simulink model "dyn_graph_sim_compact"  (R2022b)
settings: Solver=VariableStepAuto  StartTime=0.0  StopTime=100  RelTol=1e-3
values from neighbouring files (symbols this model uses):
  A = [0 1 0; 0 0 1; 0 0 -1/tau]    [cacc_consensus_main.m]    (also in dyn_graph.m; dyn_graph_10.m; dyn_graph_10_disturb.m; fixed_graph.m)
  B = [0 0 1/tau]'    [cacc_consensus_main.m]    (also in dyn_graph.m; dyn_graph_10.m; dyn_graph_10_disturb.m; fixed_graph.m)
  C = diag([1 1 1])    [cacc_consensus_main.m]    (also in dyn_graph.m; dyn_graph_10.m; dyn_graph_10_disturb.m; fixed_graph.m)
  D = [0 0 0]'    [cacc_consensus_main.m]    (also in dyn_graph.m; dyn_graph_10.m; dyn_graph_10_disturb.m; fixed_graph.m)
  h = 1    [cacc_consensus_main.m]    (also in dyn_graph.m; dyn_graph_10.m; dyn_graph_10_disturb.m; fixed_graph.m)
  K_cacc1 = [2.3231, 2.3783, -0.3394]    [dyn_graph.m]    (also in dyn_graph_10.m = -K_lmi; dyn_graph_10_disturb.m = -K_lmi; string_stability_test.m)
  K_cacc2 = [ 19.3466, 17.8329, 1.8423]    [dyn_graph.m]    (also in dyn_graph_10.m = -K_lmi; dyn_graph_10_disturb.m = -K_lmi)
  L1 = [0 0 0 0 ... (first row only)    [dyn_graph.m]    (also in dyn_graph_10.m = [0 0 0 0 0 0 0 0 0 0 0; dyn_graph_10_disturb.m = [0 0 0 0 0 0 0 0 0 0 0)
  L2 = [0 0 0 0 ... (first row only)    [dyn_graph.m]    (also in dyn_graph_10.m = [0 0 0 0 0 0 0 0 0 0 0; dyn_graph_10_disturb.m = [0 0 0 0 0 0 0 0 0 0 0)
  lv = 4.46    [cacc_consensus_main.m]    (also in dyn_graph.m; dyn_graph_10.m; dyn_graph_10_disturb.m; fixed_graph.m)
  q0_init = 0    [cacc_consensus_main.m]    (also in dyn_graph.m; dyn_graph_10.m = rand() * range; dyn_graph_10_disturb.m = rand() * range; fixed_graph.m = rand() * range)
  q1_init = 0    [cacc_consensus_main.m]    (also in dyn_graph.m; dyn_graph_10.m = rand() * range; dyn_graph_10_disturb.m = rand() * range; fixed_graph.m = rand() * range)
  q2_init = 0    [cacc_consensus_main.m]    (also in dyn_graph.m; dyn_graph_10.m = rand() * range; dyn_graph_10_disturb.m = rand() * range; fixed_graph.m = rand() * range)
  q3_init = 0    [cacc_consensus_main.m]    (also in dyn_graph.m; dyn_graph_10.m = rand() * range; dyn_graph_10_disturb.m = rand() * range; fixed_graph.m = rand() * range)
  q4_init = rand() * range    [dyn_graph_10.m]    (also in dyn_graph_10_disturb.m; fixed_graph.m; fixed_graph_lpv.m)
  q5_init = rand() * range    [dyn_graph_10.m]    (also in dyn_graph_10_disturb.m; fixed_graph.m; fixed_graph_lpv.m)
  q6_init = rand() * range    [dyn_graph_10.m]    (also in dyn_graph_10_disturb.m; fixed_graph.m; fixed_graph_lpv.m)
  q7_init = rand() * range    [dyn_graph_10.m]    (also in dyn_graph_10_disturb.m; fixed_graph.m; fixed_graph_lpv.m)
  rv = 0    [cacc_consensus_main.m]    (also in dyn_graph.m; dyn_graph_10.m; dyn_graph_10_disturb.m; fixed_graph.m)
  tau = 0.1    [cacc_consensus_main.m]    (also in dyn_graph.m; dyn_graph_10.m; dyn_graph_10_disturb.m; fixed_graph.m)
libraries: cstblocks x11, simulink x2
settings Model: Creator=phatdo  LastModifiedBy=phatdo
settings DataIOCC: ReturnWorkspaceOutputs=off

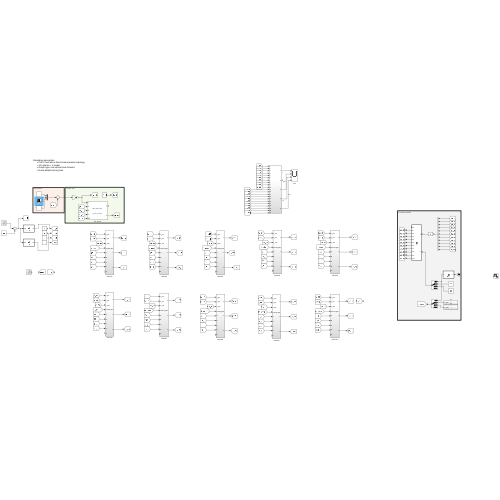
[thumbnail: Simulink's stored preview of the top-level diagram]
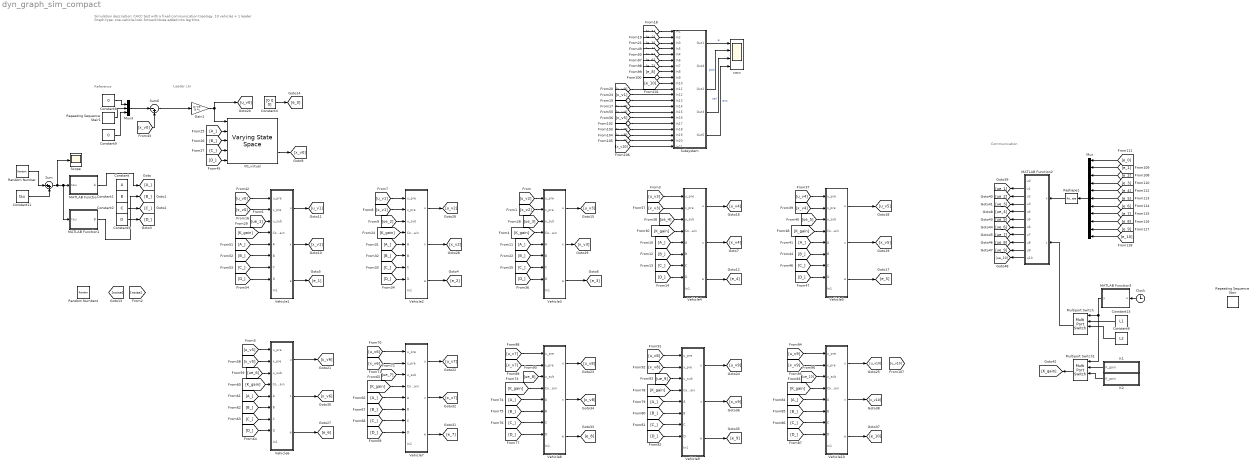
== system dyn_graph_sim_compact ==
  note: Reference
  note: Leader car
  note: Simulation description:
      | CACC test with a fixed communication topology.
      | 10 vehicles + 1 leader
      | Graph type: one-vehicle-look-forward
      | Noise added into lag time
  note: Communication
  Clock : Clock
  Constant : Constant  Value=A
  Constant1 : Constant  Value=B
  Constant11 : Constant  Value=tau
  Constant13 : Constant  Value=L1
  Constant2 : Constant  Value=C
  Constant3 : Constant  Value=D
  Constant4 : Constant  Value=[0 0 0]
  Constant6 : Constant  Value=L2
  Constant8 : Constant  Value=0
  Constant9 : Constant  Value=0
  Gain1 : Gain  Gain=[0 -0.5 0]  Multiplication=Matrix(K*u) (u vector)
  K1 : Subsystem
  K2 : Subsystem
  MATLAB Function : MATLAB Function  TreatAsAtomicUnit=on
  MATLAB Function1 : MATLAB Function  TreatAsAtomicUnit=on
  MATLAB Function2 : MATLAB Function  TreatAsAtomicUnit=on
  MATLAB Function3 : MATLAB Function  TreatAsAtomicUnit=on
  Multiport Switch : MultiPortSwitch  SaturateOnIntegerOverflow=off  InputSameDT=off
  Multiport Switch1 : MultiPortSwitch  SaturateOnIntegerOverflow=off  InputSameDT=off
  Mux : Mux  Inputs=11
  Mux3 : Mux  Inputs=3
  Random Number : RandomNumber  Variance=0.0001  SampleTime=0.1
  Random Number4 : RandomNumber  Variance=0.1  SampleTime=0.1
  Repeating Sequence Stair : simulink/Sources/Repeating Sequence Stair  OutValues=[2 1].'  tsamp=30  OutMin=[]  OutMax=[]  OutDataTypeStr=double  OutputDataTypeScalingMode=double  OutDataType=fixdt(0,8)  ConRadixGroup=Best Precision: Vector-wise  OutScaling=2^-12
  Repeating Sequence Stair1 : simulink/Sources/Repeating Sequence Stair  OutValues=[5 5 5 25 25 25 5 5 5 5]  tsamp=10  OutMin=[]  OutMax=[]  OutDataTypeStr=double  OutputDataTypeScalingMode=double  OutDataType=fixdt(0,8)  ConRadixGroup=Best Precision: Vector-wise  OutScaling=2^-12
  Reshape1 : Reshape  OutputDimensionality=Customize  OutputDimensions=[3,11]
  Scope : Scope
  Subsystem : Subsystem
  Sum : Sum  Inputs=|++
  Sum6 : Sum  Inputs=|-+
  V0_virtual : cstblocks/Linear Parameter Varying/Varying State Space  x0=[q0_init;0;0]  xNames=''  OutputX=on  OutputDX=off
  Vehicle1 : Subsystem
  Vehicle10 : Subsystem
  Vehicle2 : Subsystem
  Vehicle3 : Subsystem
  Vehicle4 : Subsystem
  Vehicle5 : Subsystem
  Vehicle6 : Subsystem
  Vehicle7 : Subsystem
  Vehicle8 : Subsystem
  Vehicle9 : Subsystem
  cacc : Scope  NumInputPorts=4
  wires:
  Constant2/1 -> [C_]
  Constant3/1 -> [D_]
  Repeating Sequence Stair1/1 -> Mux3/2
  [D_] -> V0_virtual/5
  V0_virtual/2 -> [x_v0]
  [B_] -> V0_virtual/3
  [A_] -> V0_virtual/2
  Constant9/1 -> Mux3/3
  Constant8/1 -> Mux3/1
  [x_v0] -> Sum6/2
  [C_] -> V0_virtual/4
  Sum6/1 -> Gain1/1
  Gain1/1 -> V0_virtual/1, [u_v0]
  Mux3/1 -> Sum6/1
  Sum/1 -> Scope/1, MATLAB Function1/1(tau), MATLAB Function/1(tau)
  Constant11/1 -> Sum/2
  Random Number/1 -> Sum/1
  MATLAB Function/1(A) -> [A_]
  MATLAB Function1/1(B) -> [B_]
  [u_v0] -> Vehicle1/1(u_pre)
  [K_gain] -> Vehicle1/4(Control gain)
  [A_] -> Vehicle1/5(A)
  [B_] -> Vehicle1/6(B)
  [C_] -> Vehicle1/7(C)
  [x_v0] -> Vehicle1/2(x_pre)
  [D_] -> Vehicle1/8(D)
  Vehicle1/1(u) -> [u_v1]
  Vehicle1/2(x) -> [x_v1]
  Vehicle1/3(e) -> [e_1]
  Constant4/1 -> [e_0]
  [u_v1] -> Vehicle2/1(u_pre)
  [x_v1] -> Vehicle2/2(x_pre)
  Vehicle2/3(e) -> [e_2]
  Vehicle2/2(x) -> [x_v2]
  Vehicle2/1(u) -> [u_v2]
  [K_gain] -> Vehicle2/4(Control gain)
  [A_] -> Vehicle2/5(A)
  [B_] -> Vehicle2/6(B)
  [C_] -> Vehicle2/7(C)
  [D_] -> Vehicle2/8(D)
  Vehicle3/2(x) -> [x_v3]
  [u_v2] -> Vehicle3/1(u_pre)
  [x_v2] -> Vehicle3/2(x_pre)
  Vehicle3/3(e) -> [e_3]
  [K_gain] -> Vehicle3/4(Control gain)
  [A_] -> Vehicle3/5(A)
  [B_] -> Vehicle3/6(B)
  [C_] -> Vehicle3/7(C)
  [D_] -> Vehicle3/8(D)
  Vehicle4/2(x) -> [x_v4]
  [u_v3] -> Vehicle4/1(u_pre)
  [x_v3] -> Vehicle4/2(x_pre)
  [B_] -> Vehicle4/6(B)
  [K_gain] -> Vehicle4/4(Control gain)
  [D_] -> Vehicle4/8(D)
  Vehicle4/3(e) -> [e_4]
  [C_] -> Vehicle4/7(C)
  [A_] -> Vehicle4/5(A)
  Vehicle3/1(u) -> [u_v3]
  Vehicle4/1(u) -> [u_v4]
  [u_v4] -> Vehicle5/1(u_pre)
  [x_v4] -> Vehicle5/2(x_pre)
  Vehicle5/3(e) -> [e_5]
  [K_gain] -> Vehicle5/4(Control gain)
  [A_] -> Vehicle5/5(A)
  [B_] -> Vehicle5/6(B)
  [C_] -> Vehicle5/7(C)
  [D_] -> Vehicle5/8(D)
  Vehicle5/2(x) -> [x_v5]
  Vehicle6/1(u) -> [u_v6]
  Vehicle7/1(u) -> [u_v7]
  Vehicle5/1(u) -> [u_v5]
  Vehicle8/1(u) -> [u_v8]
  Vehicle9/1(u) -> [u_v9]
  Vehicle10/1(u) -> [u_v10]
  [u_v5] -> Vehicle6/1(u_pre)
  [x_v5] -> Vehicle6/2(x_pre)
  Vehicle6/3(e) -> [e_6]
  Vehicle6/2(x) -> [x_v6]
  [K_gain] -> Vehicle6/4(Control gain)
  [A_] -> Vehicle6/5(A)
  [B_] -> Vehicle6/6(B)
  [C_] -> Vehicle6/7(C)
  [D_] -> Vehicle6/8(D)
  [K_gain] -> Vehicle7/4(Control gain)
  [A_] -> Vehicle7/5(A)
  [B_] -> Vehicle7/6(B)
  [C_] -> Vehicle7/7(C)
  [D_] -> Vehicle7/8(D)
  [u_v6] -> Vehicle7/1(u_pre)
  [x_v6] -> Vehicle7/2(x_pre)
  Vehicle7/3(e) -> [e_7]
  Vehicle7/2(x) -> [x_v7]
  Vehicle8/2(x) -> [x_v8]
  Vehicle9/2(x) -> [x_v9]
  Vehicle10/2(x) -> [x_v10]
  Vehicle10/3(e) -> [e_10]
  Vehicle9/3(e) -> [e_9]
  Vehicle8/3(e) -> [e_8]
  [K_gain] -> Vehicle8/4(Control gain)
  [A_] -> Vehicle8/5(A)
  [B_] -> Vehicle8/6(B)
  [C_] -> Vehicle8/7(C)
  [D_] -> Vehicle8/8(D)
  [K_gain] -> Vehicle9/4(Control gain)
  [A_] -> Vehicle9/5(A)
  [B_] -> Vehicle9/6(B)
  [C_] -> Vehicle9/7(C)
  [D_] -> Vehicle9/8(D)
  [K_gain] -> Vehicle10/4(Control gain)
  [A_] -> Vehicle10/5(A)
  [B_] -> Vehicle10/6(B)
  [C_] -> Vehicle10/7(C)
  [D_] -> Vehicle10/8(D)
  [u_v7] -> Vehicle8/1(u_pre)
  [x_v7] -> Vehicle8/2(x_pre)
  [u_v8] -> Vehicle9/1(u_pre)
  [x_v8] -> Vehicle9/2(x_pre)
  [u_v9] -> Vehicle10/1(u_pre)
  [x_v9] -> Vehicle10/2(x_pre)
  Multiport Switch1/1 -> [K_gain]
  MATLAB Function2/3(u2) -> [ue_2]
  [e_2] -> Mux/3
  [e_1] -> Mux/2
  Reshape1/1 -> MATLAB Function2/1(x)
  [e_0] -> Mux/1
  Multiport Switch/1 -> MATLAB Function2/2(L)
  Constant6/1 -> Multiport Switch/3
  Constant13/1 -> Multiport Switch/2
  Mux/1 -> Reshape1/1
  MATLAB Function2/2(u1) -> [ue_1]
  MATLAB Function2/4(u3) -> [ue_3]
  [e_3] -> Mux/4
  MATLAB Function2/5(u4) -> [ue_4]
  MATLAB Function2/6(u5) -> [ue_5]
  MATLAB Function2/7(u6) -> [ue_6]
  MATLAB Function2/8(u7) -> [ue_7]
  MATLAB Function2/9(u8) -> [ue_8]
  MATLAB Function2/10(u9) -> [ue_9]
  MATLAB Function2/11(u10) -> [ue_10]
  [e_4] -> Mux/5
  [e_5] -> Mux/6
  [e_6] -> Mux/7
  [e_7] -> Mux/8
  [e_8] -> Mux/9
  [e_9] -> Mux/10
  [e_10] -> Mux/11
  [ue_10] -> Vehicle10/3(u_sub)
  [ue_9] -> Vehicle9/3(u_sub)
  [ue_8] -> Vehicle8/3(u_sub)
  [ue_7] -> Vehicle7/3(u_sub)
  [ue_6] -> Vehicle6/3(u_sub)
  [ue_5] -> Vehicle5/3(u_sub)
  [ue_4] -> Vehicle4/3(u_sub)
  [ue_3] -> Vehicle3/3(u_sub)
  [ue_2] -> Vehicle2/3(u_sub)
  [ue_1] -> Vehicle1/3(u_sub)
  Clock/1 -> MATLAB Function3/1(u)
  MATLAB Function3/1(y) -> Multiport Switch1/1, Multiport Switch/1
  K1/1(K_gain) -> Multiport Switch1/2
  K2/1(K_gain) -> Multiport Switch1/3
  [x_v0] -> Subsystem/11(In11)
  [x_v5] -> Subsystem/16(In16)
  [x_v9] -> Subsystem/20(In20)
  Subsystem/1(Out1) -> cacc/1  "e"
  [x_v10] -> Subsystem/21(In21)
  [e_10] -> Subsystem/10(In10)
  [e_9] -> Subsystem/9(In9)
  [e_7] -> Subsystem/7(In7)
  [e_6] -> Subsystem/6(In6)
  [x_v8] -> Subsystem/19(In19)
  [e_8] -> Subsystem/8(In8)
  [x_v7] -> Subsystem/18(In18)
  [x_v2] -> Subsystem/13(In13)
  [e_1] -> Subsystem/1(In1)
  [x_v6] -> Subsystem/17(In17)
  [e_4] -> Subsystem/4(In5)
  [x_v3] -> Subsystem/14(In14)
  Subsystem/5(Out5) -> cacc/4  "acc"
  [x_v1] -> Subsystem/12(In12)
  Subsystem/4(Out3) -> cacc/3  "vel"
  [e_3] -> Subsystem/3(In3)
  Subsystem/3(Out2) -> cacc/2  "pos"
  [e_5] -> Subsystem/5(In4)
  [x_v4] -> Subsystem/15(In15)
  [e_2] -> Subsystem/2(In2)

== system dyn_graph_sim_compact/K1 ==
  Constant : Constant
  K1 : Fcn  Expr=-K_cacc1(2)
  K2 : Fcn  Expr=0
  K4 : Fcn  Expr=-K_cacc1(1)
  Mux : Mux  Inputs=3
  Reshape : Reshape  OutputDimensionality=Customize  OutputDimensions=[1,3]
  K_gain : Outport
  wires:
  Mux/1 -> Reshape/1
  Reshape/1 -> K_gain/1
  K4/1 -> Mux/1
  K1/1 -> Mux/2
  K2/1 -> Mux/3
  Constant/1 -> K2/1, K1/1, K4/1

== system dyn_graph_sim_compact/K2 ==
  Constant : Constant
  K1 : Fcn  Expr=-K_cacc2(2)
  K2 : Fcn  Expr=0
  K4 : Fcn  Expr=-K_cacc2(1)
  Mux : Mux  Inputs=3
  Reshape : Reshape  OutputDimensionality=Customize  OutputDimensions=[1,3]
  K_gain : Outport
  wires:
  Mux/1 -> Reshape/1
  Reshape/1 -> K_gain/1
  K4/1 -> Mux/1
  K1/1 -> Mux/2
  K2/1 -> Mux/3
  Constant/1 -> K2/1, K1/1, K4/1

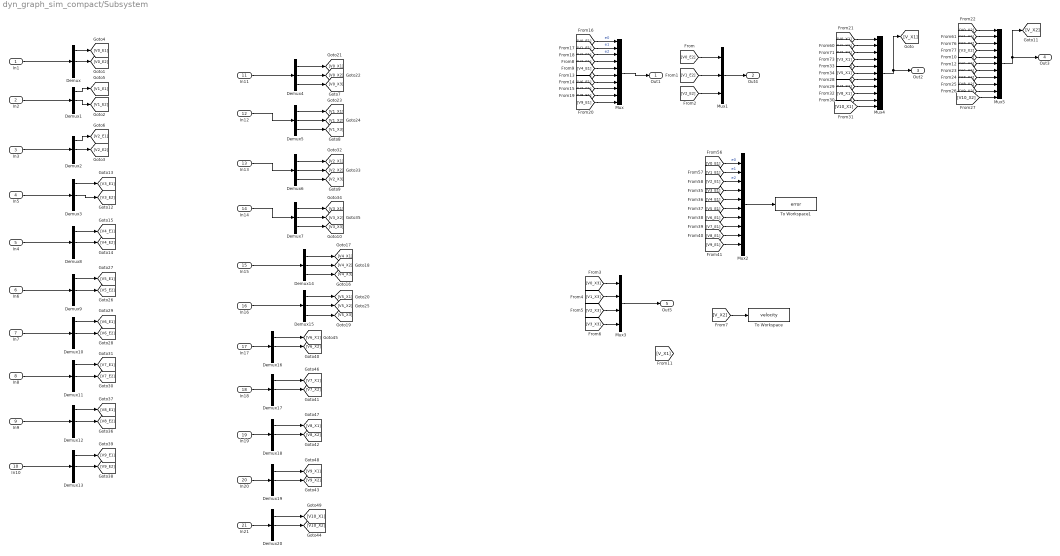
== system dyn_graph_sim_compact/Subsystem ==
  In1 : Inport
  In2 : Inport  Port=2
  In3 : Inport  Port=3
  In5 : Inport  Port=4
  In4 : Inport  Port=5
  In6 : Inport  Port=6
  In7 : Inport  Port=7
  In8 : Inport  Port=8
  In9 : Inport  Port=9
  In10 : Inport  Port=10
  In11 : Inport  Port=11
  In12 : Inport  Port=12
  In13 : Inport  Port=13
  In14 : Inport  Port=14
  In15 : Inport  Port=15
  In16 : Inport  Port=16
  In17 : Inport  Port=17
  In18 : Inport  Port=18
  In19 : Inport  Port=19
  In20 : Inport  Port=20
  In21 : Inport  Port=21
  Demux{,1..20} (21 alike) : Demux  Outputs=3
  Mux : Mux  Inputs=10
  Mux1 : Mux  Inputs=3
  Mux2 : Mux  Inputs=10
  Mux3 : Mux
  Mux4 : Mux  Inputs=11
  Mux5 : Mux  Inputs=11
  To Workspace : ToWorkspace  VariableName=velocity  SaveFormat=Timeseries  SampleTime=-1
  To Workspace1 : ToWorkspace  VariableName=error  SaveFormat=Timeseries  SampleTime=-1
  Out1 : Outport
  Out4 : Outport  Port=2
  Out2 : Outport  Port=3
  Out3 : Outport  Port=4
  Out5 : Outport  Port=5
  wires:
  [V2_X1] -> Mux4/3
  Demux/1 -> [V0_E1]
  Demux2/1 -> [V2_E1]
  In2/1 -> Demux1/1
  [V0_X1] -> Mux4/1
  Demux1/1 -> [V1_E1]
  [V3_X1] -> Mux4/4
  Demux6/2 -> [V2_X2]
  Demux7/1 -> [V3_X1]
  Demux4/1 -> [V0_X1]
  Demux4/2 -> [V0_X2]
  Demux5/2 -> [V1_X2]
  Demux6/1 -> [V2_X1]
  [V1_X2] -> Mux5/2
  In1/1 -> Demux/1
  Mux4/1 -> [V_X1], Out2/1
  [V3_X2] -> Mux5/4
  [V2_X2] -> Mux5/3
  [V0_X2] -> Mux5/1
  Demux7/2 -> [V3_X2]
  [V1_E1] -> Mux/2  "e1"
  [V1_X1] -> Mux4/2
  [V2_E1] -> Mux/3  "e2"
  [V0_E1] -> Mux/1  "e0"
  Mux/1 -> Out1/1
  In3/1 -> Demux2/1
  Demux5/1 -> [V1_X1]
  Demux/2 -> [V0_E2]
  Demux1/2 -> [V1_E2]
  Demux2/2 -> [V2_E2]
  [V0_E2] -> Mux1/1
  [V1_E2] -> Mux1/2
  [V2_E2] -> Mux1/3
  Mux1/1 -> Out4/1
  Demux4/3 -> [V0_X3]
  Demux5/3 -> [V1_X3]
  Demux6/3 -> [V2_X3]
  Demux7/3 -> [V3_X3]
  [V0_X3] -> Mux3/1
  [V1_X3] -> Mux3/2
  [V2_X3] -> Mux3/3
  [V3_X3] -> Mux3/4
  Mux3/1 -> Out5/1
  Mux5/1 -> [V_X2], Out3/1
  In5/1 -> Demux3/1
  In4/1 -> Demux8/1
  In6/1 -> Demux9/1
  In7/1 -> Demux10/1
  In8/1 -> Demux11/1
  In9/1 -> Demux12/1
  In10/1 -> Demux13/1
  In11/1 -> Demux4/1
  In12/1 -> Demux5/1
  In13/1 -> Demux6/1
  In14/1 -> Demux7/1
  Demux3/1 -> [V3_E1]
  Demux8/1 -> [V4_E1]
  Demux3/2 -> [V3_E2]
  Demux8/2 -> [V4_E2]
  Demux14/1 -> [V4_X1]
  In15/1 -> Demux14/1
  Demux14/2 -> [V4_X2]
  Demux14/3 -> [V4_X3]
  Demux15/1 -> [V5_X1]
  In16/1 -> Demux15/1
  Demux15/2 -> [V5_X2]
  Demux15/3 -> [V5_X3]
  [V3_E1] -> Mux/4
  [V4_E1] -> Mux/5
  [V4_X2] -> Mux5/5
  [V5_X2] -> Mux5/6
  Demux9/1 -> [V5_E1]
  Demux9/2 -> [V5_E2]
  Demux10/1 -> [V6_E1]
  Demux10/2 -> [V6_E2]
  Demux11/1 -> [V7_E1]
  Demux11/2 -> [V7_E2]
  Demux12/1 -> [V8_E1]
  Demux12/2 -> [V8_E2]
  Demux13/1 -> [V9_E1]
  Demux13/2 -> [V9_E2]
  [V5_E1] -> Mux/6
  [V6_E1] -> Mux/7
  [V7_E1] -> Mux/8
  [V8_E1] -> Mux/9
  [V9_E1] -> Mux/10
  Demux16/2 -> [V6_X2]
  Demux17/2 -> [V7_X2]
  Demux18/2 -> [V8_X2]
  Demux19/2 -> [V9_X2]
  Demux20/2 -> [V10_X2]
  In17/1 -> Demux16/1
  In18/1 -> Demux17/1
  In19/1 -> Demux18/1
  In20/1 -> Demux19/1
  In21/1 -> Demux20/1
  [V6_X2] -> Mux5/7
  [V7_X2] -> Mux5/8
  [V8_X2] -> Mux5/9
  [V9_X2] -> Mux5/10
  [V10_X2] -> Mux5/11
  Demux16/1 -> [V6_X1]
  Demux17/1 -> [V7_X1]
  Demux18/1 -> [V8_X1]
  Demux19/1 -> [V9_X1]
  Demux20/1 -> [V10_X1]
  [V4_X1] -> Mux4/5
  [V5_X1] -> Mux4/6
  [V6_X1] -> Mux4/7
  [V7_X1] -> Mux4/8
  [V8_X1] -> Mux4/9
  [V9_X1] -> Mux4/10
  [V10_X1] -> Mux4/11
  [V_X2] -> To Workspace/1
  [V0_E1] -> Mux2/1  "e0"
  [V1_E1] -> Mux2/2  "e1"
  [V2_E1] -> Mux2/3  "e2"
  [V3_E1] -> Mux2/4
  [V4_E1] -> Mux2/5
  [V5_E1] -> Mux2/6
  [V6_E1] -> Mux2/7
  [V7_E1] -> Mux2/8
  [V8_E1] -> Mux2/9
  [V9_E1] -> Mux2/10
  Mux2/1 -> To Workspace1/1

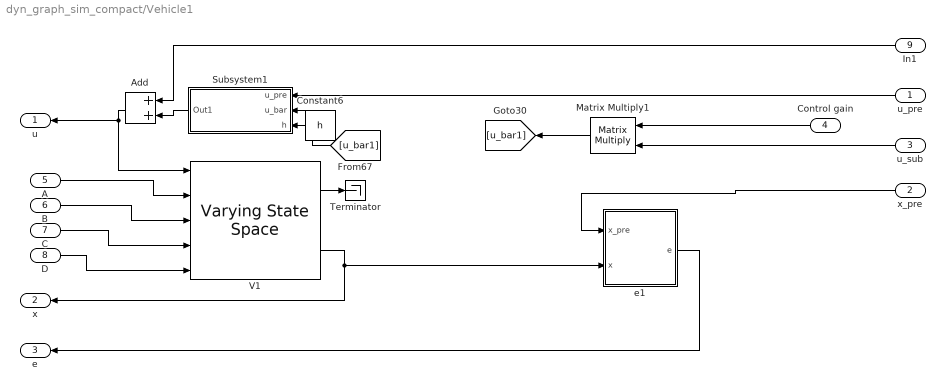
== system dyn_graph_sim_compact/Vehicle1 ==
  u_pre : Inport
  x_pre : Inport  Port=2
  u_sub : Inport  Port=3
  Control gain : Inport  Port=4
  A : Inport  Port=5
  B : Inport  Port=6
  C : Inport  Port=7
  D : Inport  Port=8
  In1 : Inport  Port=9
  Add : Sum
  Constant6 : Constant  Value=h
  Matrix Multiply1 : Product  Multiplication=Matrix(*)
  Subsystem1 : Subsystem
  Terminator : Terminator
  V1 : cstblocks/Linear Parameter Varying/Varying State Space  x0=[q1_init;0;0]  xNames=''  OutputX=on  OutputDX=off
  e1 : Subsystem
  u : Outport
  x : Outport  Port=2
  e : Outport  Port=3
  wires:
  C/1 -> V1/4
  Matrix Multiply1/1 -> [u_bar1]
  Constant6/1 -> Subsystem1/3(h)
  x_pre/1 -> e1/1(x_pre)
  e1/1(e) -> e/1
  Control gain/1 -> Matrix Multiply1/1
  D/1 -> V1/5
  B/1 -> V1/3
  A/1 -> V1/2
  In1/1 -> Add/1
  Add/1 -> u/1, V1/1
  V1/1 -> Terminator/1
  V1/2 -> x/1, e1/2(x)
  Subsystem1/1(Out1) -> Add/2
  [u_bar1] -> Subsystem1/2(u_bar)
  u_pre/1 -> Subsystem1/1(u_pre)
  u_sub/1 -> Matrix Multiply1/2

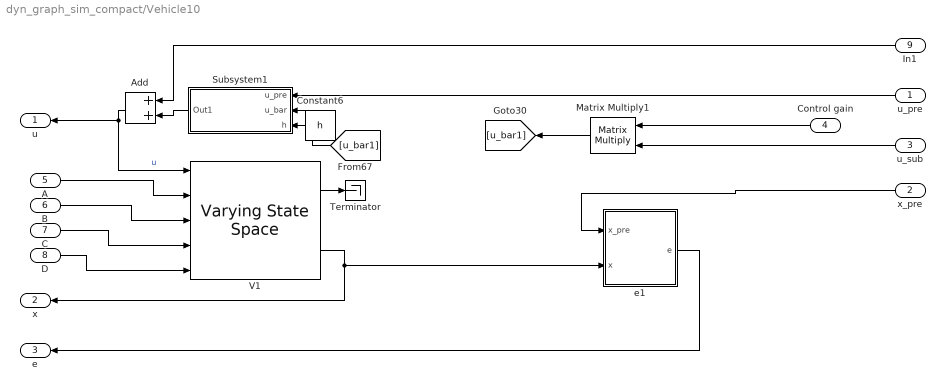
== system dyn_graph_sim_compact/Vehicle10 ==
  u_pre : Inport
  x_pre : Inport  Port=2
  u_sub : Inport  Port=3
  Control gain : Inport  Port=4
  A : Inport  Port=5
  B : Inport  Port=6
  C : Inport  Port=7
  D : Inport  Port=8
  In1 : Inport  Port=9
  Add : Sum
  Constant6 : Constant  Value=h
  Matrix Multiply1 : Product  Multiplication=Matrix(*)
  Subsystem1 : Subsystem
  Terminator : Terminator
  V1 : cstblocks/Linear Parameter Varying/Varying State Space  x0=[q5_init;0;0]  xNames=''  OutputX=on  OutputDX=off
  e1 : Subsystem
  u : Outport
  x : Outport  Port=2
  e : Outport  Port=3
  wires:
  C/1 -> V1/4
  Matrix Multiply1/1 -> [u_bar1]
  Constant6/1 -> Subsystem1/3(h)
  x_pre/1 -> e1/1(x_pre)
  e1/1(e) -> e/1
  Control gain/1 -> Matrix Multiply1/1
  D/1 -> V1/5
  B/1 -> V1/3
  A/1 -> V1/2
  In1/1 -> Add/1
  Add/1 -> u/1, V1/1  "u"
  V1/1 -> Terminator/1
  V1/2 -> x/1, e1/2(x)
  Subsystem1/1(Out1) -> Add/2
  [u_bar1] -> Subsystem1/2(u_bar)
  u_pre/1 -> Subsystem1/1(u_pre)
  u_sub/1 -> Matrix Multiply1/2

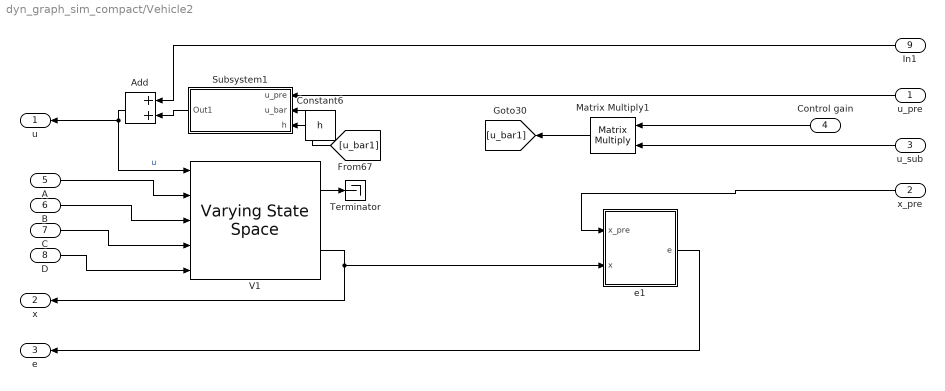
== system dyn_graph_sim_compact/Vehicle2 ==
  u_pre : Inport
  x_pre : Inport  Port=2
  u_sub : Inport  Port=3
  Control gain : Inport  Port=4
  A : Inport  Port=5
  B : Inport  Port=6
  C : Inport  Port=7
  D : Inport  Port=8
  In1 : Inport  Port=9
  Add : Sum
  Constant6 : Constant  Value=h
  Matrix Multiply1 : Product  Multiplication=Matrix(*)
  Subsystem1 : Subsystem
  Terminator : Terminator
  V1 : cstblocks/Linear Parameter Varying/Varying State Space  x0=[q2_init;0;0]  xNames=''  OutputX=on  OutputDX=off
  e1 : Subsystem
  u : Outport
  x : Outport  Port=2
  e : Outport  Port=3
  wires:
  C/1 -> V1/4
  Matrix Multiply1/1 -> [u_bar1]
  Constant6/1 -> Subsystem1/3(h)
  x_pre/1 -> e1/1(x_pre)
  e1/1(e) -> e/1
  Control gain/1 -> Matrix Multiply1/1
  D/1 -> V1/5
  B/1 -> V1/3
  A/1 -> V1/2
  In1/1 -> Add/1
  Add/1 -> u/1, V1/1  "u"
  V1/1 -> Terminator/1
  V1/2 -> x/1, e1/2(x)
  Subsystem1/1(Out1) -> Add/2
  [u_bar1] -> Subsystem1/2(u_bar)
  u_pre/1 -> Subsystem1/1(u_pre)
  u_sub/1 -> Matrix Multiply1/2

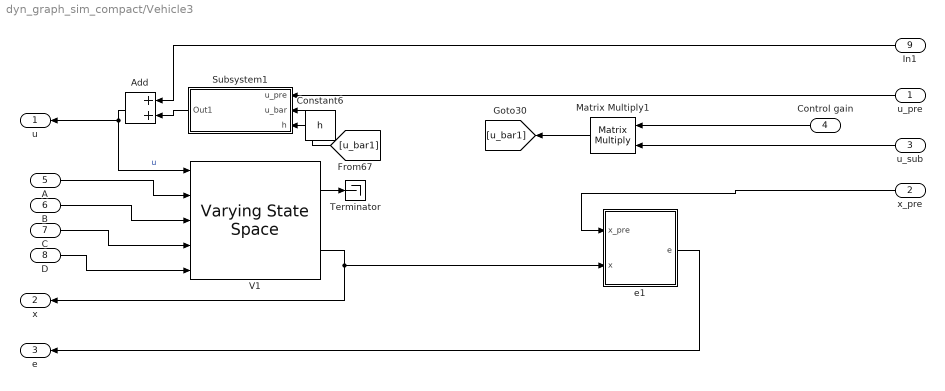
== system dyn_graph_sim_compact/Vehicle3 ==
  u_pre : Inport
  x_pre : Inport  Port=2
  u_sub : Inport  Port=3
  Control gain : Inport  Port=4
  A : Inport  Port=5
  B : Inport  Port=6
  C : Inport  Port=7
  D : Inport  Port=8
  In1 : Inport  Port=9
  Add : Sum
  Constant6 : Constant  Value=h
  Matrix Multiply1 : Product  Multiplication=Matrix(*)
  Subsystem1 : Subsystem
  Terminator : Terminator
  V1 : cstblocks/Linear Parameter Varying/Varying State Space  x0=[q3_init;0;0]  xNames=''  OutputX=on  OutputDX=off
  e1 : Subsystem
  u : Outport
  x : Outport  Port=2
  e : Outport  Port=3
  wires:
  C/1 -> V1/4
  Matrix Multiply1/1 -> [u_bar1]
  Constant6/1 -> Subsystem1/3(h)
  x_pre/1 -> e1/1(x_pre)
  e1/1(e) -> e/1
  Control gain/1 -> Matrix Multiply1/1
  D/1 -> V1/5
  B/1 -> V1/3
  A/1 -> V1/2
  In1/1 -> Add/1
  Add/1 -> u/1, V1/1  "u"
  V1/1 -> Terminator/1
  V1/2 -> x/1, e1/2(x)
  Subsystem1/1(Out1) -> Add/2
  [u_bar1] -> Subsystem1/2(u_bar)
  u_pre/1 -> Subsystem1/1(u_pre)
  u_sub/1 -> Matrix Multiply1/2

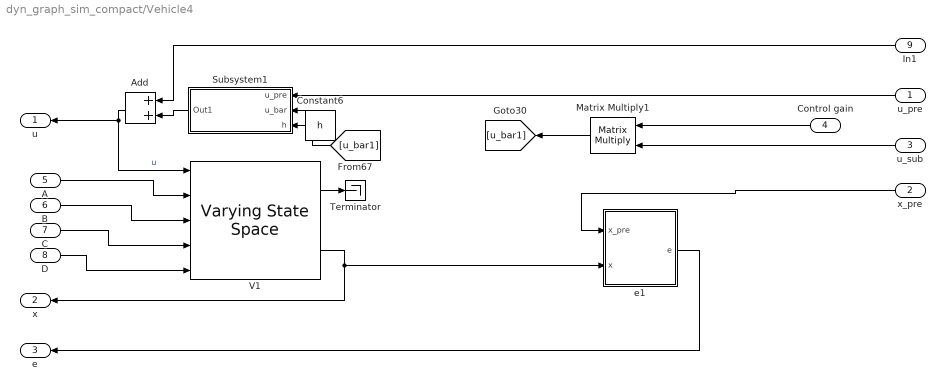
== system dyn_graph_sim_compact/Vehicle4 ==
  u_pre : Inport
  x_pre : Inport  Port=2
  u_sub : Inport  Port=3
  Control gain : Inport  Port=4
  A : Inport  Port=5
  B : Inport  Port=6
  C : Inport  Port=7
  D : Inport  Port=8
  In1 : Inport  Port=9
  Add : Sum
  Constant6 : Constant  Value=h
  Matrix Multiply1 : Product  Multiplication=Matrix(*)
  Subsystem1 : Subsystem
  Terminator : Terminator
  V1 : cstblocks/Linear Parameter Varying/Varying State Space  x0=[q4_init;0;0]  xNames=''  OutputX=on  OutputDX=off
  e1 : Subsystem
  u : Outport
  x : Outport  Port=2
  e : Outport  Port=3
  wires:
  C/1 -> V1/4
  Matrix Multiply1/1 -> [u_bar1]
  Constant6/1 -> Subsystem1/3(h)
  x_pre/1 -> e1/1(x_pre)
  e1/1(e) -> e/1
  Control gain/1 -> Matrix Multiply1/1
  D/1 -> V1/5
  B/1 -> V1/3
  A/1 -> V1/2
  In1/1 -> Add/1
  Add/1 -> u/1, V1/1  "u"
  V1/1 -> Terminator/1
  V1/2 -> x/1, e1/2(x)
  Subsystem1/1(Out1) -> Add/2
  [u_bar1] -> Subsystem1/2(u_bar)
  u_pre/1 -> Subsystem1/1(u_pre)
  u_sub/1 -> Matrix Multiply1/2

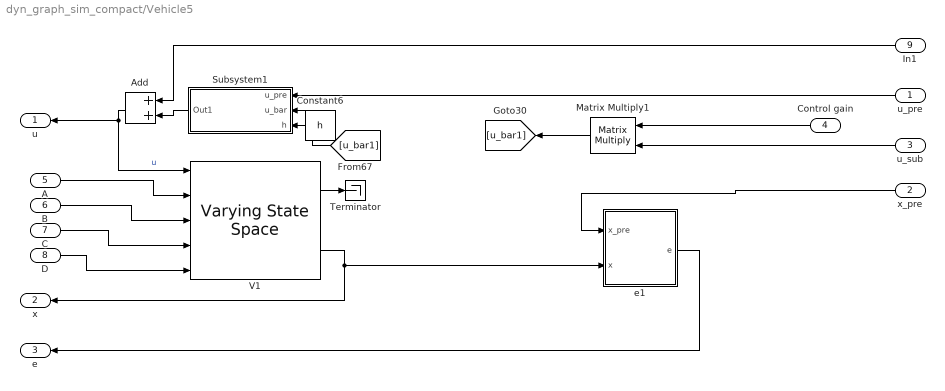
== system dyn_graph_sim_compact/Vehicle5 ==
  u_pre : Inport
  x_pre : Inport  Port=2
  u_sub : Inport  Port=3
  Control gain : Inport  Port=4
  A : Inport  Port=5
  B : Inport  Port=6
  C : Inport  Port=7
  D : Inport  Port=8
  In1 : Inport  Port=9
  Add : Sum
  Constant6 : Constant  Value=h
  Matrix Multiply1 : Product  Multiplication=Matrix(*)
  Subsystem1 : Subsystem
  Terminator : Terminator
  V1 : cstblocks/Linear Parameter Varying/Varying State Space  x0=[q5_init;0;0]  xNames=''  OutputX=on  OutputDX=off
  e1 : Subsystem
  u : Outport
  x : Outport  Port=2
  e : Outport  Port=3
  wires:
  C/1 -> V1/4
  Matrix Multiply1/1 -> [u_bar1]
  Constant6/1 -> Subsystem1/3(h)
  x_pre/1 -> e1/1(x_pre)
  e1/1(e) -> e/1
  Control gain/1 -> Matrix Multiply1/1
  D/1 -> V1/5
  B/1 -> V1/3
  A/1 -> V1/2
  In1/1 -> Add/1
  Add/1 -> u/1, V1/1  "u"
  V1/1 -> Terminator/1
  V1/2 -> x/1, e1/2(x)
  Subsystem1/1(Out1) -> Add/2
  [u_bar1] -> Subsystem1/2(u_bar)
  u_pre/1 -> Subsystem1/1(u_pre)
  u_sub/1 -> Matrix Multiply1/2

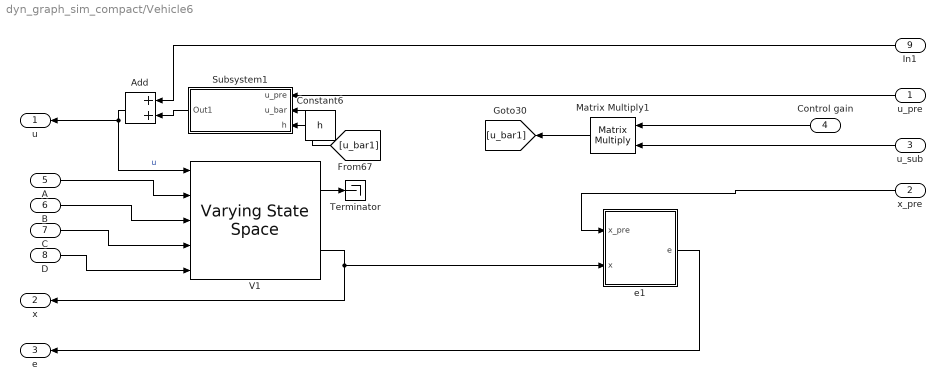
== system dyn_graph_sim_compact/Vehicle6 ==
  u_pre : Inport
  x_pre : Inport  Port=2
  u_sub : Inport  Port=3
  Control gain : Inport  Port=4
  A : Inport  Port=5
  B : Inport  Port=6
  C : Inport  Port=7
  D : Inport  Port=8
  In1 : Inport  Port=9
  Add : Sum
  Constant6 : Constant  Value=h
  Matrix Multiply1 : Product  Multiplication=Matrix(*)
  Subsystem1 : Subsystem
  Terminator : Terminator
  V1 : cstblocks/Linear Parameter Varying/Varying State Space  x0=[q6_init;0;0]  xNames=''  OutputX=on  OutputDX=off
  e1 : Subsystem
  u : Outport
  x : Outport  Port=2
  e : Outport  Port=3
  wires:
  C/1 -> V1/4
  Matrix Multiply1/1 -> [u_bar1]
  Constant6/1 -> Subsystem1/3(h)
  x_pre/1 -> e1/1(x_pre)
  e1/1(e) -> e/1
  Control gain/1 -> Matrix Multiply1/1
  D/1 -> V1/5
  B/1 -> V1/3
  A/1 -> V1/2
  In1/1 -> Add/1
  Add/1 -> u/1, V1/1  "u"
  V1/1 -> Terminator/1
  V1/2 -> x/1, e1/2(x)
  Subsystem1/1(Out1) -> Add/2
  [u_bar1] -> Subsystem1/2(u_bar)
  u_pre/1 -> Subsystem1/1(u_pre)
  u_sub/1 -> Matrix Multiply1/2

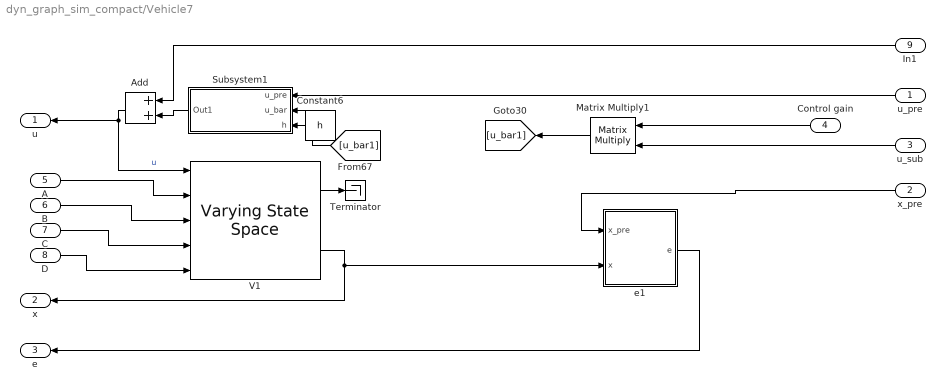
== system dyn_graph_sim_compact/Vehicle7 ==
  u_pre : Inport
  x_pre : Inport  Port=2
  u_sub : Inport  Port=3
  Control gain : Inport  Port=4
  A : Inport  Port=5
  B : Inport  Port=6
  C : Inport  Port=7
  D : Inport  Port=8
  In1 : Inport  Port=9
  Add : Sum
  Constant6 : Constant  Value=h
  Matrix Multiply1 : Product  Multiplication=Matrix(*)
  Subsystem1 : Subsystem
  Terminator : Terminator
  V1 : cstblocks/Linear Parameter Varying/Varying State Space  x0=[q7_init;0;0]  xNames=''  OutputX=on  OutputDX=off
  e1 : Subsystem
  u : Outport
  x : Outport  Port=2
  e : Outport  Port=3
  wires:
  C/1 -> V1/4
  Matrix Multiply1/1 -> [u_bar1]
  Constant6/1 -> Subsystem1/3(h)
  x_pre/1 -> e1/1(x_pre)
  e1/1(e) -> e/1
  Control gain/1 -> Matrix Multiply1/1
  D/1 -> V1/5
  B/1 -> V1/3
  A/1 -> V1/2
  In1/1 -> Add/1
  Add/1 -> u/1, V1/1  "u"
  V1/1 -> Terminator/1
  V1/2 -> x/1, e1/2(x)
  Subsystem1/1(Out1) -> Add/2
  [u_bar1] -> Subsystem1/2(u_bar)
  u_pre/1 -> Subsystem1/1(u_pre)
  u_sub/1 -> Matrix Multiply1/2

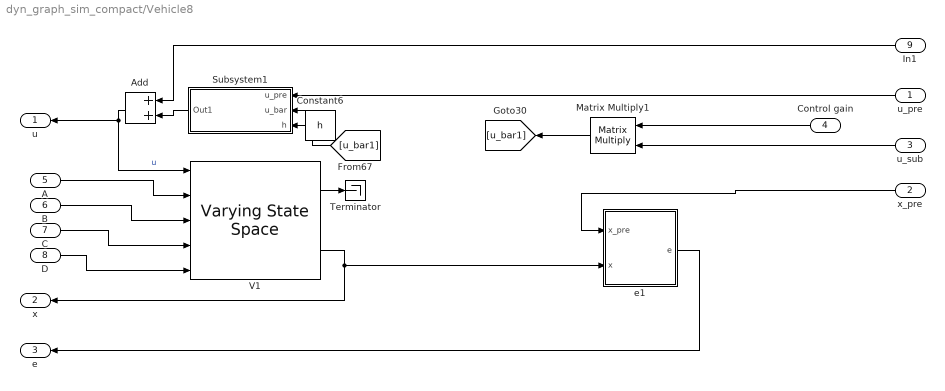
== system dyn_graph_sim_compact/Vehicle8 ==
  u_pre : Inport
  x_pre : Inport  Port=2
  u_sub : Inport  Port=3
  Control gain : Inport  Port=4
  A : Inport  Port=5
  B : Inport  Port=6
  C : Inport  Port=7
  D : Inport  Port=8
  In1 : Inport  Port=9
  Add : Sum
  Constant6 : Constant  Value=h
  Matrix Multiply1 : Product  Multiplication=Matrix(*)
  Subsystem1 : Subsystem
  Terminator : Terminator
  V1 : cstblocks/Linear Parameter Varying/Varying State Space  x0=[q5_init;0;0]  xNames=''  OutputX=on  OutputDX=off
  e1 : Subsystem
  u : Outport
  x : Outport  Port=2
  e : Outport  Port=3
  wires:
  C/1 -> V1/4
  Matrix Multiply1/1 -> [u_bar1]
  Constant6/1 -> Subsystem1/3(h)
  x_pre/1 -> e1/1(x_pre)
  e1/1(e) -> e/1
  Control gain/1 -> Matrix Multiply1/1
  D/1 -> V1/5
  B/1 -> V1/3
  A/1 -> V1/2
  In1/1 -> Add/1
  Add/1 -> u/1, V1/1  "u"
  V1/1 -> Terminator/1
  V1/2 -> x/1, e1/2(x)
  Subsystem1/1(Out1) -> Add/2
  [u_bar1] -> Subsystem1/2(u_bar)
  u_pre/1 -> Subsystem1/1(u_pre)
  u_sub/1 -> Matrix Multiply1/2

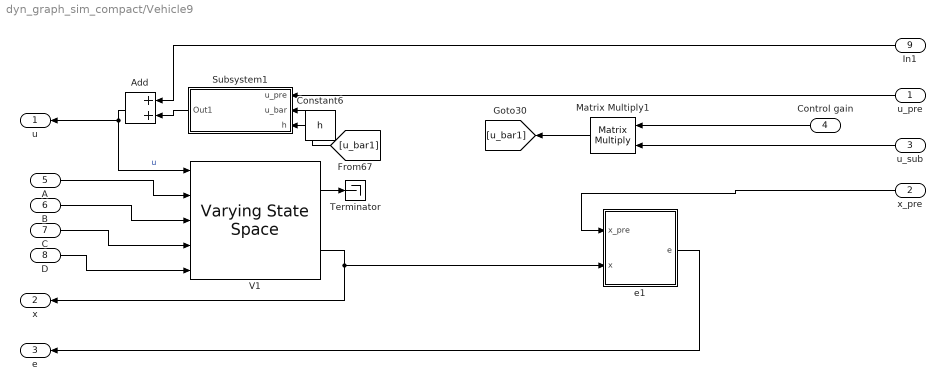
== system dyn_graph_sim_compact/Vehicle9 ==
  u_pre : Inport
  x_pre : Inport  Port=2
  u_sub : Inport  Port=3
  Control gain : Inport  Port=4
  A : Inport  Port=5
  B : Inport  Port=6
  C : Inport  Port=7
  D : Inport  Port=8
  In1 : Inport  Port=9
  Add : Sum
  Constant6 : Constant  Value=h
  Matrix Multiply1 : Product  Multiplication=Matrix(*)
  Subsystem1 : Subsystem
  Terminator : Terminator
  V1 : cstblocks/Linear Parameter Varying/Varying State Space  x0=[q5_init;0;0]  xNames=''  OutputX=on  OutputDX=off
  e1 : Subsystem
  u : Outport
  x : Outport  Port=2
  e : Outport  Port=3
  wires:
  C/1 -> V1/4
  Matrix Multiply1/1 -> [u_bar1]
  Constant6/1 -> Subsystem1/3(h)
  x_pre/1 -> e1/1(x_pre)
  e1/1(e) -> e/1
  Control gain/1 -> Matrix Multiply1/1
  D/1 -> V1/5
  B/1 -> V1/3
  A/1 -> V1/2
  In1/1 -> Add/1
  Add/1 -> u/1, V1/1  "u"
  V1/1 -> Terminator/1
  V1/2 -> x/1, e1/2(x)
  Subsystem1/1(Out1) -> Add/2
  [u_bar1] -> Subsystem1/2(u_bar)
  u_pre/1 -> Subsystem1/1(u_pre)
  u_sub/1 -> Matrix Multiply1/2

== system dyn_graph_sim_compact/Vehicle1/Subsystem1 ==
  u_pre : Inport
  u_bar : Inport  Port=2
  h : Inport  Port=3
  Controller dyn : MATLAB Function  TreatAsAtomicUnit=on
  Integrator : Integrator
  Out1 : Outport
  wires:
  Controller dyn/1(u_dot) -> Integrator/1
  Integrator/1 -> Controller dyn/1(u), Out1/1
  u_pre/1 -> Controller dyn/2(u_pre)
  u_bar/1 -> Controller dyn/3(u_bar)
  h/1 -> Controller dyn/4(h)

== system dyn_graph_sim_compact/Vehicle1/e1 ==
  x_pre : Inport
  x : Inport  Port=2
  " " : Demux  Outputs=3
  "   " : Demux  Outputs=3
  Constant : Constant  Value=0
  Gain : Gain  Gain=h
  Gain1 : Gain  Gain=h
  Mux : Mux  Inputs=3
  Sum : Sum  Inputs=|+----
  Sum1 : Sum  Inputs=|+--
  lv : Constant  Value=lv
  rv : Constant  Value=rv
  e : Outport
  wires:
  " "/1 -> Sum/1
  "   "/1 -> Sum/2
  lv/1 -> Sum/3
  rv/1 -> Sum/4
  Gain/1 -> Sum/5
  Sum/1 -> Mux/1
  "   "/2 -> Sum1/2, Gain/1
  " "/2 -> Sum1/1
  "   "/3 -> Gain1/1
  Gain1/1 -> Sum1/3
  x_pre/1 -> " "/1
  x/1 -> "   "/1
  Constant/1 -> Mux/3
  Mux/1 -> e/1
  Sum1/1 -> Mux/2

== system dyn_graph_sim_compact/Vehicle10/Subsystem1 ==
  u_pre : Inport
  u_bar : Inport  Port=2
  h : Inport  Port=3
  Controller dyn : MATLAB Function  TreatAsAtomicUnit=on
  Integrator : Integrator
  Out1 : Outport
  wires:
  Controller dyn/1(u_dot) -> Integrator/1
  Integrator/1 -> Controller dyn/1(u), Out1/1
  u_pre/1 -> Controller dyn/2(u_pre)
  u_bar/1 -> Controller dyn/3(u_bar)
  h/1 -> Controller dyn/4(h)

== system dyn_graph_sim_compact/Vehicle10/e1 ==
  x_pre : Inport
  x : Inport  Port=2
  " " : Demux  Outputs=3
  "   " : Demux  Outputs=3
  Constant : Constant  Value=0
  Gain : Gain  Gain=h
  Gain1 : Gain  Gain=h
  Mux : Mux  Inputs=3
  Sum : Sum  Inputs=|+----
  Sum1 : Sum  Inputs=|+--
  lv : Constant  Value=lv
  rv : Constant  Value=rv
  e : Outport
  wires:
  " "/1 -> Sum/1
  "   "/1 -> Sum/2
  lv/1 -> Sum/3
  rv/1 -> Sum/4
  Gain/1 -> Sum/5
  Sum/1 -> Mux/1
  "   "/2 -> Sum1/2, Gain/1
  " "/2 -> Sum1/1
  "   "/3 -> Gain1/1
  Gain1/1 -> Sum1/3
  x_pre/1 -> " "/1
  x/1 -> "   "/1
  Constant/1 -> Mux/3
  Mux/1 -> e/1
  Sum1/1 -> Mux/2

== system dyn_graph_sim_compact/Vehicle2/Subsystem1 ==
  u_pre : Inport
  u_bar : Inport  Port=2
  h : Inport  Port=3
  Controller dyn : MATLAB Function  TreatAsAtomicUnit=on
  Integrator : Integrator
  Out1 : Outport
  wires:
  Controller dyn/1(u_dot) -> Integrator/1
  Integrator/1 -> Controller dyn/1(u), Out1/1
  u_pre/1 -> Controller dyn/2(u_pre)
  u_bar/1 -> Controller dyn/3(u_bar)
  h/1 -> Controller dyn/4(h)

== system dyn_graph_sim_compact/Vehicle2/e1 ==
  x_pre : Inport
  x : Inport  Port=2
  " " : Demux  Outputs=3
  "   " : Demux  Outputs=3
  Constant : Constant  Value=0
  Gain : Gain  Gain=h
  Gain1 : Gain  Gain=h
  Mux : Mux  Inputs=3
  Sum : Sum  Inputs=|+----
  Sum1 : Sum  Inputs=|+--
  lv : Constant  Value=lv
  rv : Constant  Value=rv
  e : Outport
  wires:
  " "/1 -> Sum/1
  "   "/1 -> Sum/2
  lv/1 -> Sum/3
  rv/1 -> Sum/4
  Gain/1 -> Sum/5
  Sum/1 -> Mux/1
  "   "/2 -> Sum1/2, Gain/1
  " "/2 -> Sum1/1
  "   "/3 -> Gain1/1
  Gain1/1 -> Sum1/3
  x_pre/1 -> " "/1
  x/1 -> "   "/1
  Constant/1 -> Mux/3
  Mux/1 -> e/1
  Sum1/1 -> Mux/2

== system dyn_graph_sim_compact/Vehicle3/Subsystem1 ==
  u_pre : Inport
  u_bar : Inport  Port=2
  h : Inport  Port=3
  Controller dyn : MATLAB Function  TreatAsAtomicUnit=on
  Integrator : Integrator
  Out1 : Outport
  wires:
  Controller dyn/1(u_dot) -> Integrator/1
  Integrator/1 -> Controller dyn/1(u), Out1/1
  u_pre/1 -> Controller dyn/2(u_pre)
  u_bar/1 -> Controller dyn/3(u_bar)
  h/1 -> Controller dyn/4(h)

== system dyn_graph_sim_compact/Vehicle3/e1 ==
  x_pre : Inport
  x : Inport  Port=2
  " " : Demux  Outputs=3
  "   " : Demux  Outputs=3
  Constant : Constant  Value=0
  Gain : Gain  Gain=h
  Gain1 : Gain  Gain=h
  Mux : Mux  Inputs=3
  Sum : Sum  Inputs=|+----
  Sum1 : Sum  Inputs=|+--
  lv : Constant  Value=lv
  rv : Constant  Value=rv
  e : Outport
  wires:
  " "/1 -> Sum/1
  "   "/1 -> Sum/2
  lv/1 -> Sum/3
  rv/1 -> Sum/4
  Gain/1 -> Sum/5
  Sum/1 -> Mux/1
  "   "/2 -> Sum1/2, Gain/1
  " "/2 -> Sum1/1
  "   "/3 -> Gain1/1
  Gain1/1 -> Sum1/3
  x_pre/1 -> " "/1
  x/1 -> "   "/1
  Constant/1 -> Mux/3
  Mux/1 -> e/1
  Sum1/1 -> Mux/2

== system dyn_graph_sim_compact/Vehicle4/Subsystem1 ==
  u_pre : Inport
  u_bar : Inport  Port=2
  h : Inport  Port=3
  Controller dyn : MATLAB Function  TreatAsAtomicUnit=on
  Integrator : Integrator
  Out1 : Outport
  wires:
  Controller dyn/1(u_dot) -> Integrator/1
  Integrator/1 -> Controller dyn/1(u), Out1/1
  u_pre/1 -> Controller dyn/2(u_pre)
  u_bar/1 -> Controller dyn/3(u_bar)
  h/1 -> Controller dyn/4(h)

== system dyn_graph_sim_compact/Vehicle4/e1 ==
  x_pre : Inport
  x : Inport  Port=2
  " " : Demux  Outputs=3
  "   " : Demux  Outputs=3
  Constant : Constant  Value=0
  Gain : Gain  Gain=h
  Gain1 : Gain  Gain=h
  Mux : Mux  Inputs=3
  Sum : Sum  Inputs=|+----
  Sum1 : Sum  Inputs=|+--
  lv : Constant  Value=lv
  rv : Constant  Value=rv
  e : Outport
  wires:
  " "/1 -> Sum/1
  "   "/1 -> Sum/2
  lv/1 -> Sum/3
  rv/1 -> Sum/4
  Gain/1 -> Sum/5
  Sum/1 -> Mux/1
  "   "/2 -> Sum1/2, Gain/1
  " "/2 -> Sum1/1
  "   "/3 -> Gain1/1
  Gain1/1 -> Sum1/3
  x_pre/1 -> " "/1
  x/1 -> "   "/1
  Constant/1 -> Mux/3
  Mux/1 -> e/1
  Sum1/1 -> Mux/2

== system dyn_graph_sim_compact/Vehicle5/Subsystem1 ==
  u_pre : Inport
  u_bar : Inport  Port=2
  h : Inport  Port=3
  Controller dyn : MATLAB Function  TreatAsAtomicUnit=on
  Integrator : Integrator
  Out1 : Outport
  wires:
  Controller dyn/1(u_dot) -> Integrator/1
  Integrator/1 -> Controller dyn/1(u), Out1/1
  u_pre/1 -> Controller dyn/2(u_pre)
  u_bar/1 -> Controller dyn/3(u_bar)
  h/1 -> Controller dyn/4(h)

== system dyn_graph_sim_compact/Vehicle5/e1 ==
  x_pre : Inport
  x : Inport  Port=2
  " " : Demux  Outputs=3
  "   " : Demux  Outputs=3
  Constant : Constant  Value=0
  Gain : Gain  Gain=h
  Gain1 : Gain  Gain=h
  Mux : Mux  Inputs=3
  Sum : Sum  Inputs=|+----
  Sum1 : Sum  Inputs=|+--
  lv : Constant  Value=lv
  rv : Constant  Value=rv
  e : Outport
  wires:
  " "/1 -> Sum/1
  "   "/1 -> Sum/2
  lv/1 -> Sum/3
  rv/1 -> Sum/4
  Gain/1 -> Sum/5
  Sum/1 -> Mux/1
  "   "/2 -> Sum1/2, Gain/1
  " "/2 -> Sum1/1
  "   "/3 -> Gain1/1
  Gain1/1 -> Sum1/3
  x_pre/1 -> " "/1
  x/1 -> "   "/1
  Constant/1 -> Mux/3
  Mux/1 -> e/1
  Sum1/1 -> Mux/2

== system dyn_graph_sim_compact/Vehicle6/Subsystem1 ==
  u_pre : Inport
  u_bar : Inport  Port=2
  h : Inport  Port=3
  Controller dyn : MATLAB Function  TreatAsAtomicUnit=on
  Integrator : Integrator
  Out1 : Outport
  wires:
  Controller dyn/1(u_dot) -> Integrator/1
  Integrator/1 -> Controller dyn/1(u), Out1/1
  u_pre/1 -> Controller dyn/2(u_pre)
  u_bar/1 -> Controller dyn/3(u_bar)
  h/1 -> Controller dyn/4(h)

== system dyn_graph_sim_compact/Vehicle6/e1 ==
  x_pre : Inport
  x : Inport  Port=2
  " " : Demux  Outputs=3
  "   " : Demux  Outputs=3
  Constant : Constant  Value=0
  Gain : Gain  Gain=h
  Gain1 : Gain  Gain=h
  Mux : Mux  Inputs=3
  Sum : Sum  Inputs=|+----
  Sum1 : Sum  Inputs=|+--
  lv : Constant  Value=lv
  rv : Constant  Value=rv
  e : Outport
  wires:
  " "/1 -> Sum/1
  "   "/1 -> Sum/2
  lv/1 -> Sum/3
  rv/1 -> Sum/4
  Gain/1 -> Sum/5
  Sum/1 -> Mux/1
  "   "/2 -> Sum1/2, Gain/1
  " "/2 -> Sum1/1
  "   "/3 -> Gain1/1
  Gain1/1 -> Sum1/3
  x_pre/1 -> " "/1
  x/1 -> "   "/1
  Constant/1 -> Mux/3
  Mux/1 -> e/1
  Sum1/1 -> Mux/2

== system dyn_graph_sim_compact/Vehicle7/Subsystem1 ==
  u_pre : Inport
  u_bar : Inport  Port=2
  h : Inport  Port=3
  Controller dyn : MATLAB Function  TreatAsAtomicUnit=on
  Integrator : Integrator
  Out1 : Outport
  wires:
  Controller dyn/1(u_dot) -> Integrator/1
  Integrator/1 -> Controller dyn/1(u), Out1/1
  u_pre/1 -> Controller dyn/2(u_pre)
  u_bar/1 -> Controller dyn/3(u_bar)
  h/1 -> Controller dyn/4(h)

== system dyn_graph_sim_compact/Vehicle7/e1 ==
  x_pre : Inport
  x : Inport  Port=2
  " " : Demux  Outputs=3
  "   " : Demux  Outputs=3
  Constant : Constant  Value=0
  Gain : Gain  Gain=h
  Gain1 : Gain  Gain=h
  Mux : Mux  Inputs=3
  Sum : Sum  Inputs=|+----
  Sum1 : Sum  Inputs=|+--
  lv : Constant  Value=lv
  rv : Constant  Value=rv
  e : Outport
  wires:
  " "/1 -> Sum/1
  "   "/1 -> Sum/2
  lv/1 -> Sum/3
  rv/1 -> Sum/4
  Gain/1 -> Sum/5
  Sum/1 -> Mux/1
  "   "/2 -> Sum1/2, Gain/1
  " "/2 -> Sum1/1
  "   "/3 -> Gain1/1
  Gain1/1 -> Sum1/3
  x_pre/1 -> " "/1
  x/1 -> "   "/1
  Constant/1 -> Mux/3
  Mux/1 -> e/1
  Sum1/1 -> Mux/2

== system dyn_graph_sim_compact/Vehicle8/Subsystem1 ==
  u_pre : Inport
  u_bar : Inport  Port=2
  h : Inport  Port=3
  Controller dyn : MATLAB Function  TreatAsAtomicUnit=on
  Integrator : Integrator
  Out1 : Outport
  wires:
  Controller dyn/1(u_dot) -> Integrator/1
  Integrator/1 -> Controller dyn/1(u), Out1/1
  u_pre/1 -> Controller dyn/2(u_pre)
  u_bar/1 -> Controller dyn/3(u_bar)
  h/1 -> Controller dyn/4(h)

== system dyn_graph_sim_compact/Vehicle8/e1 ==
  x_pre : Inport
  x : Inport  Port=2
  " " : Demux  Outputs=3
  "   " : Demux  Outputs=3
  Constant : Constant  Value=0
  Gain : Gain  Gain=h
  Gain1 : Gain  Gain=h
  Mux : Mux  Inputs=3
  Sum : Sum  Inputs=|+----
  Sum1 : Sum  Inputs=|+--
  lv : Constant  Value=lv
  rv : Constant  Value=rv
  e : Outport
  wires:
  " "/1 -> Sum/1
  "   "/1 -> Sum/2
  lv/1 -> Sum/3
  rv/1 -> Sum/4
  Gain/1 -> Sum/5
  Sum/1 -> Mux/1
  "   "/2 -> Sum1/2, Gain/1
  " "/2 -> Sum1/1
  "   "/3 -> Gain1/1
  Gain1/1 -> Sum1/3
  x_pre/1 -> " "/1
  x/1 -> "   "/1
  Constant/1 -> Mux/3
  Mux/1 -> e/1
  Sum1/1 -> Mux/2

== system dyn_graph_sim_compact/Vehicle9/Subsystem1 ==
  u_pre : Inport
  u_bar : Inport  Port=2
  h : Inport  Port=3
  Controller dyn : MATLAB Function  TreatAsAtomicUnit=on
  Integrator : Integrator
  Out1 : Outport
  wires:
  Controller dyn/1(u_dot) -> Integrator/1
  Integrator/1 -> Controller dyn/1(u), Out1/1
  u_pre/1 -> Controller dyn/2(u_pre)
  u_bar/1 -> Controller dyn/3(u_bar)
  h/1 -> Controller dyn/4(h)

== system dyn_graph_sim_compact/Vehicle9/e1 ==
  x_pre : Inport
  x : Inport  Port=2
  " " : Demux  Outputs=3
  "   " : Demux  Outputs=3
  Constant : Constant  Value=0
  Gain : Gain  Gain=h
  Gain1 : Gain  Gain=h
  Mux : Mux  Inputs=3
  Sum : Sum  Inputs=|+----
  Sum1 : Sum  Inputs=|+--
  lv : Constant  Value=lv
  rv : Constant  Value=rv
  e : Outport
  wires:
  " "/1 -> Sum/1
  "   "/1 -> Sum/2
  lv/1 -> Sum/3
  rv/1 -> Sum/4
  Gain/1 -> Sum/5
  Sum/1 -> Mux/1
  "   "/2 -> Sum1/2, Gain/1
  " "/2 -> Sum1/1
  "   "/3 -> Gain1/1
  Gain1/1 -> Sum1/3
  x_pre/1 -> " "/1
  x/1 -> "   "/1
  Constant/1 -> Mux/3
  Mux/1 -> e/1
  Sum1/1 -> Mux/2

== matlab function dyn_graph_sim_compact/Vehicle8/Subsystem1/Controller dyn ==
  data: u input; u_dot output; u_pre input; u_bar input; h input
function u_dot = cacc(u, u_pre, u_bar,h)

h = h; % second

u_dot = -1/h * u + 1/h * (u_pre - u_bar);

end

== matlab function dyn_graph_sim_compact/Vehicle9/Subsystem1/Controller dyn ==
  data: u input; u_dot output; u_pre input; u_bar input; h input
function u_dot = cacc(u, u_pre, u_bar,h)

h = h; % second

u_dot = -1/h * u + 1/h * (u_pre - u_bar);

end

== matlab function dyn_graph_sim_compact/Vehicle10/Subsystem1/Controller dyn ==
  data: u input; u_dot output; u_pre input; u_bar input; h input
function u_dot = cacc(u, u_pre, u_bar,h)

h = h; % second

u_dot = -1/h * u + 1/h * (u_pre - u_bar);

end

== matlab function dyn_graph_sim_compact/MATLAB Function2 ==
  data: x input; L input; u0 output; u1 output; u2 output; u3 output; u4 output; u5 output; u6 output; u7 output; u8 output; u9 output; u10 output
function [u0,u1,u2,u3,u4,u5,u6,u7,u8,u9,u10] = fcn(x, L)

n = length(L);
uk = zeros(length(x(:,1)),1);
u = uk;
for i = 1:n
    uk = zeros(length(x(:,1)),1);
    for j = 1:n
    uk = uk + L(i,j)*x(:,j);
    end
    if i == 1
        u = uk;
    else
        u = [u uk];
    end
end
u0 = (u(:,1));
u1 = (u(:,2));
u2 = (u(:,3));
u3 = (u(:,4));
u4 = (u(:,5));
u5 = (u(:,6));
u6 = (u(:,7));
u7 = (u(:,8));
u8 = (u(:,9));
u9 = (u(:,10));
u10 = (u(:,11));
end

== matlab function dyn_graph_sim_compact/MATLAB Function3 ==
  data: u input; y output
function y = fcn(u)
if u < 30
    y = 2;
else
    y = 2;
end
end

== matlab function dyn_graph_sim_compact/Vehicle1/Subsystem1/Controller dyn ==
  data: u input; u_dot output; u_pre input; u_bar input; h input
function u_dot = cacc(u, u_pre, u_bar,h)

h = h; % second

u_dot = -1/h * u + 1/h * (u_pre - u_bar);

end

== matlab function dyn_graph_sim_compact/MATLAB Function ==
  data: tau input; A output
function A = fcn(tau)

A = [0 1 0; 0 0 1; 0 0 -1/tau];

end

== matlab function dyn_graph_sim_compact/Vehicle3/Subsystem1/Controller dyn ==
  data: u input; u_dot output; u_pre input; u_bar input; h input
function u_dot = cacc(u, u_pre, u_bar,h)

h = h; % second

u_dot = -1/h * u + 1/h * (u_pre - u_bar);

end

== matlab function dyn_graph_sim_compact/MATLAB Function1 ==
  data: tau input; B output
function B = fcn(tau)

B = [0; 0; 1/tau];

end

== matlab function dyn_graph_sim_compact/Vehicle4/Subsystem1/Controller dyn ==
  data: u input; u_dot output; u_pre input; u_bar input; h input
function u_dot = cacc(u, u_pre, u_bar,h)

h = h; % second

u_dot = -1/h * u + 1/h * (u_pre - u_bar);

end

== matlab function dyn_graph_sim_compact/Vehicle2/Subsystem1/Controller dyn ==
  data: u input; u_dot output; u_pre input; u_bar input; h input
function u_dot = cacc(u, u_pre, u_bar,h)

h = h; % second

u_dot = -1/h * u + 1/h * (u_pre - u_bar);

end

== matlab function dyn_graph_sim_compact/Vehicle5/Subsystem1/Controller dyn ==
  data: u input; u_dot output; u_pre input; u_bar input; h input
function u_dot = cacc(u, u_pre, u_bar,h)

h = h; % second

u_dot = -1/h * u + 1/h * (u_pre - u_bar);

end

== matlab function dyn_graph_sim_compact/Vehicle6/Subsystem1/Controller dyn ==
  data: u input; u_dot output; u_pre input; u_bar input; h input
function u_dot = cacc(u, u_pre, u_bar,h)

h = h; % second

u_dot = -1/h * u + 1/h * (u_pre - u_bar);

end

== matlab function dyn_graph_sim_compact/Vehicle7/Subsystem1/Controller dyn ==
  data: u input; u_dot output; u_pre input; u_bar input; h input
function u_dot = cacc(u, u_pre, u_bar,h)

h = h; % second

u_dot = -1/h * u + 1/h * (u_pre - u_bar);

end
